simulink model "ModelFull"  (R2023a)
settings: Solver=FixedStepAuto  StartTime=0.0  StopTime=inf  RelTol=1e-3  EnableMultiTasking=on
model workspace (MAT data in the model file):
  time = 1
values from neighbouring files (symbols this model uses):
  Deq = 0.01    [matlab.mat]
  Kmotor = 0.5    [matlab.mat]
  R = 5    [matlab.mat]
libraries: fl_lib x12, arduinolib x7, ee_lib x4, simulink x3, nesl_utility x3, arduinosensorlib x2
(part 1 of 3)
settings Model: ExtModeTrigDuration=2  Creator=Adham  LastModifiedBy=moham
settings DataIOCC: InspectSignalLogs=on
settings OptimizationCC: EnhancedBackFolding=on  PassReuseOutputArgsAs=Individual arguments  ZeroExternalMemoryAtStartup=off  ZeroInternalMemoryAtStartup=off  MaxStackSize=64  OptimizeBlockOrder=speed  DifferentSizesBufferReuse=on  OptimizationCustomize=off  EfficientTunableParamExpr=on
settings DebuggingCC: ParameterTunabilityLossMsg=error
settings HardwareCC: ProdBitPerInt=16  ProdBitPerPointer=16  ProdBitPerSizeT=16  ProdBitPerPtrDiffT=16  ProdLargestAtomicFloat=None  ProdWordSize=8  ProdHWDeviceType=Atmel->AVR  UseEmbeddedCoderFeatures=off
settings SFSimCC: MATLABDynamicMemAlloc=off
settings RTWCC: Description=Embedded Coder  SystemTargetFile=ert.tlc  HardwareBoard=Arduino Uno  TemplateMakefile=ert_default_tmf  Toolchain=Arduino AVR  BuildConfiguration=Faster Runs
settings CodeAppCC: ForceParamTrailComments=on  IgnoreCustomStorageClasses=off  OperatorAnnotations=on  SimulinkDataObjDesc=on  SFDataObjDesc=on  InsertBlockDesc=on
settings ERTTargetCC: SupportContinuousTime=on  SupportNonInlinedSFcns=on  SupportVariableSizeSignals=on  ExtModeTransport=3  ExtModeStaticAlloc=on  ExtModeAutomaticAllocSize=off  ExtModeStaticAllocSize=250  ExtModeMexFile=ext_xcp  ExtModeIntrfLevel=Level2 - Open

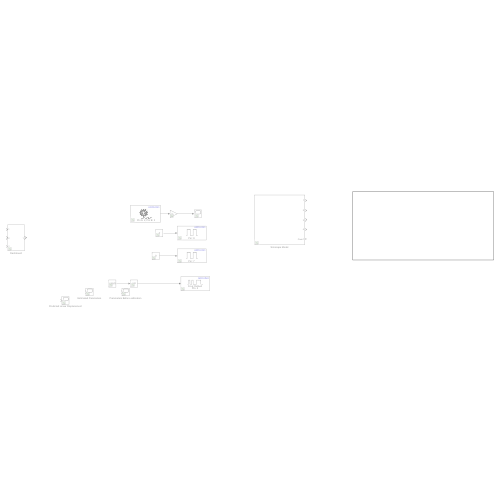
[thumbnail: Simulink's stored preview of the top-level diagram]
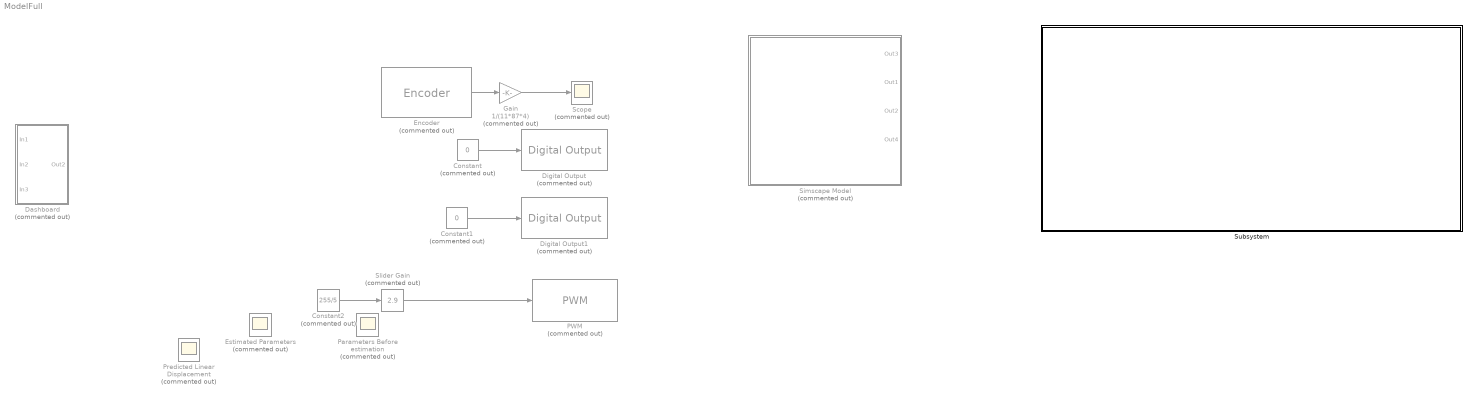
== system ModelFull ==
  Constant : Constant  Commented=on  Value=0
  Constant1 : Constant  Commented=on  Value=0
  Constant2 : Constant  Commented=on  Value=255/5
  Dashboard : Subsystem  Commented=on
  Digital Output : arduinolib/Digital Output  Commented=on  pinNumber=8  Direction=output  blockPlatform=arduino
  Digital Output1 : arduinolib/Digital Output  Commented=on  pinNumber=7  Direction=output  blockPlatform=arduino
  Encoder : arduinosensorlib/Encoder  Commented=on  InputA=2  InputB=3  Mode=No reset  SampleTime=-1
  Estimated Parameters : Scope  Commented=on
  Gain : Gain  Commented=on  Gain=1/(11*87*4)
  PWM : arduinolib/PWM  Commented=on  pinNumber=5  frequencyType=Default  desiredFrequency=490.2  achievableFrequency=490.2
  Parameters Before estimation : Scope  Commented=on
  Predicted Linear Displacement : Scope  Commented=on
  Scope : Scope  Commented=on
  Simscape Model : Subsystem  Commented=on
  Slider Gain : simulink/Math Operations/Slider Gain  Commented=on  gain=2.9  low=0  high=5
  Subsystem : Subsystem
  wires:
  Constant/1 -> Digital Output/1
  Encoder/1 -> Gain/1
  Constant2/1 -> Slider Gain/1
  Constant1/1 -> Digital Output1/1
  Gain/1 -> Scope/1
  Slider Gain/1 -> PWM/1
